simulink subsystem "Controller"  (R2021a)
settings: Solver=VariableStepAuto  StartTime=0.0  StopTime=10.0  RelTol=1e-3
values from neighbouring files (symbols this model uses):
  MPC =     [matlab.mat]
  N = [-39.9215617836 -39.7361560536 -39.4691718024 -38.8907059248 -38.267742672 -37.9562610456 -37.5112872936 -37.2888004176 -36.7993292904 -36.4433502888 -35.8648844112 -35.1974237832 ... (201 elements, 201x1)]    [matlab.mat]
  physics =     [matlab.mat]
  PWM = [1100 1104 1108 1112 1116 1120 1124 1128 1132 1136 1140 1144 ... (201 elements, 201x1)]    [matlab.mat]
libraries: mpclib x5, sharedTrackingLibrary x3, sharedtransform x2, simulink x1
settings Model: Creator=Lamarre  LastModifiedBy=lamarre
settings SolverCC: AlgebraicLoopSolver=TrustRegion
settings DebuggingCC: SFMachineParentedDataDiag=warning

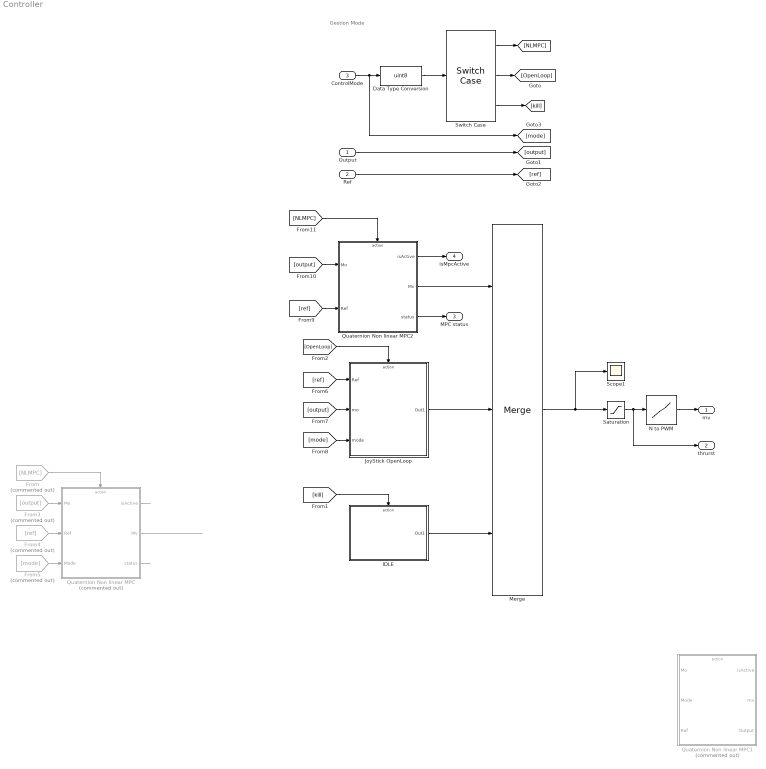
== system Controller ==
  note: Gestion Mode
  Output : Inport
  Ref : Inport  Port=2
  ControlMode : Inport  Port=3
  Data Type Conversion : DataTypeConversion  OutDataTypeStr=uint8
  From : From  Commented=on  GotoTag=NLMPC
  From3 : From  Commented=on  GotoTag=output
  From4 : From  Commented=on  GotoTag=ref
  From5 : From  Commented=on  GotoTag=mode
  IDLE : Subsystem  TreatAsAtomicUnit=on
  JoyStick OpenLoop : Subsystem  TreatAsAtomicUnit=on
  Merge : Merge  Inputs=3
  N to PWM : Lookup_n-D  NumberOfTableDimensions=1  BreakpointsForDimension1=N  BeginIndexSearchUsingPreviousIndexResult=on  Table=PWM  InterpMethod=Nearest  ExtrapMethod=Clip  DiagnosticForOutOfRangeInput=Warning  RemoveProtectionInput=on  InternalRulePriority=Speed  OutDataTypeStr=uint16  RndMeth=Simplest  InputSameDT=on
  Quaternion Non linear MPC : Subsystem  Commented=on
  Quaternion Non linear MPC1 : Subsystem  Commented=on
  Quaternion Non linear MPC2 : Subsystem
  Saturation : Saturate  UpperLimit=MPC.tmax  LowerLimit=MPC.tmin
  Scope1 : Scope
  Switch Case : SwitchCase  CaseConditions={mpcMode, openLoopMode}
  mv : Outport
  thrurst : Outport  Port=2
  MPC status : Outport  Port=3
  isMpcActive : Outport  Port=4
  wires:
  Switch Case/3 -> [kill]
  Switch Case/1 -> [NLMPC]
  N to PWM/1 -> mv/1
  [kill] -> IDLE/Action
  Data Type Conversion/1 -> Switch Case/1
  Switch Case/2 -> [OpenLoop]
  JoyStick OpenLoop/1(Out1) -> Merge/2
  IDLE/1(Out1) -> Merge/3
  [OpenLoop] -> JoyStick OpenLoop/Action
  ControlMode/1 -> Data Type Conversion/1, [mode]
  Output/1 -> [output]
  Ref/1 -> [ref]
  [ref] -> JoyStick OpenLoop/1(Ref)
  [output] -> JoyStick OpenLoop/2(mo)
  [mode] -> JoyStick OpenLoop/3(mode)
  Saturation/1 -> N to PWM/1, thrurst/1
  Merge/1 -> Scope1/1, Saturation/1
  [output] -> Quaternion Non linear MPC2/1(Mo)
  [ref] -> Quaternion Non linear MPC2/2(Ref)
  From3/1 -> Quaternion Non linear MPC/1(Mo)
  Quaternion Non linear MPC/3(status) -> ?
  From4/1 -> Quaternion Non linear MPC/2(Ref)
  From5/1 -> Quaternion Non linear MPC/3(Mode)
  Quaternion Non linear MPC/1(isActive) -> ?
  From/1 -> Quaternion Non linear MPC/Action
  Quaternion Non linear MPC/2(Mv) -> ?
  Quaternion Non linear MPC2/3(status) -> MPC status/1
  Quaternion Non linear MPC2/1(isActive) -> isMpcActive/1
  Quaternion Non linear MPC2/2(Mv) -> Merge/1
  [NLMPC] -> Quaternion Non linear MPC2/Action

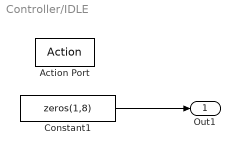
== system Controller/IDLE ==
  Action Port : ActionPort
  Constant1 : Constant  Value=zeros(1,8)
  Out1 : Outport
  wires:
  Constant1/1 -> Out1/1

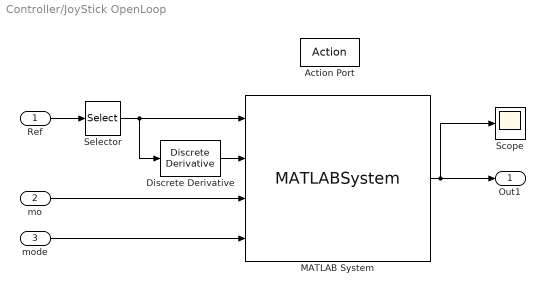
== system Controller/JoyStick OpenLoop ==
  Ref : Inport
  mo : Inport  Port=2
  mode : Inport  Port=3
  Action Port : ActionPort
  Discrete Derivative : simulink/Discrete/Discrete Derivative  gainval=1.0  ICPrevScaledInput=0.0  OutMin=[]  OutMax=[]  OutDataType=fixdt(1, 16)  OutScaling=2^-10  DoSatur=off
  MATLAB System : MATLABSystem  System=OpenLoopController  k=40  binv=binv  mass=physics.mass  volume=physics.volume  height=physics.height  I=physics.I  RG=physics.RG  RB=physics.RB  AddedMass=physics.AddedMass  CDL=physics.CDL  CDQ=physics.CDQ  AF=physics.AF  g=physics.g  rho=physics.rho  SimulateUsing=Code generation
      mask Type: OpenLoopController
      mask Display:
      | disp('OpenLoopController');
      | port_label('input',1,'ref');
      | port_label('input',2,'ref_dot');
      | port_label('input',3,'mo');
      | port_label('input',4,'mode');
      | port_label('output',1,'mv');
  Scope : Scope
  Selector : Selector  NumberOfDimensions=2  InputPortWidth=13  IndexOptions=Index vector (dialog),Index vector (dialog)  Indices=1,[8:13]  OutputSizes=1,1
  Out1 : Outport
  wires:
  Selector/1 -> MATLAB System/1, Discrete Derivative/1
  Discrete Derivative/1 -> MATLAB System/2
  Ref/1 -> Selector/1
  MATLAB System/1 -> Out1/1, Scope/1
  mode/1 -> MATLAB System/4
  mo/1 -> MATLAB System/3

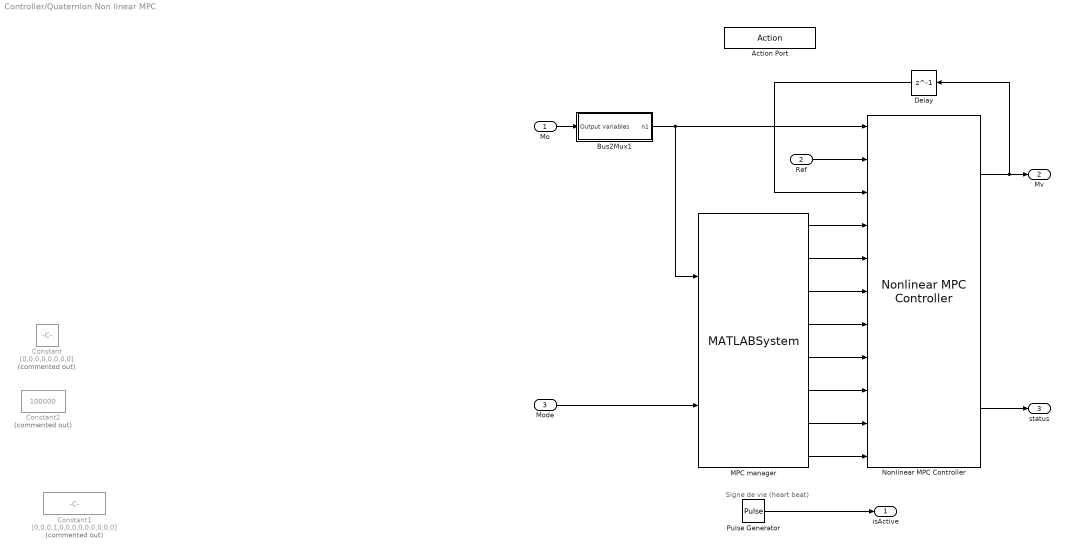
== system Controller/Quaternion Non linear MPC ==
  note: Signe de vie (heart beat)
  Mo : Inport
  Ref : Inport  Port=2
  Mode : Inport  Port=3
  Action Port : ActionPort  InitializeStates=reset
  Bus2Mux1 : Subsystem
  Constant : Constant  Commented=on  Value=[0,0,0,0,0,0,0,0]  VectorParams1D=off
  Constant1 : Constant  Commented=on  Value=[0,0,0,1,0,0,0,0,0,0,0,0,0]  VectorParams1D=off
  Constant2 : Constant  Commented=on  Value=100000
  Delay : Delay  DelayLength=1  InitialCondition=[0,0,0,0,0,0,0,0].'
  MPC manager : MATLABSystem  System=mpcManager  Config10=Config10  Config19=Config19  Tmin=ones( 1, 8 )*MPC.tmin  Tmax=ones( 1, 8 )*MPC.tmax  MecConst=constValues  mvInit=Ui  eInit=0  SimulateUsing=Code generation
      mask Type: mpcManager
      mask Display:
      | disp('mpcManager');
      | port_label('input',1,'x0');
      | port_label('input',2,'mode');
      | port_label('output',1,'mvmin');
      | port_label('output',2,'mvmax');
      | port_label('output',3,'ywt');
      | port_label('output',4,'mvwt');
      | port_label('output',5,'dmwwt');
      | port_label('output',6,'mvInit');
      | port_label('output',7,'xInit');
      | port_label('output',8,'eInit');
  Nonlinear MPC Controller : mpclib/Nonlinear MPC Controller  SCDEnableBlockLinearizationSpecification=on  nlmpcobj=nlobj  UseObjectTs=on  TsControl=mpc.Ts  UseMEX=off  md_enabled=off  mvtarget_enabled=off  param_enabled=off  cost_enabled=off  mvseq_enabled=off  stateseq_enabled=on  ovseq_enabled=off  slack_enabled=off  status_enabled=on  ov_min=off  ov_max=off  mv_min=on  mv_max=on  mvrate_min=off  mvrate_max=off  state_min=off  state_max=off  ov_weight=on  mv_weight=on  mvrate_weight=on  ecr_weight=off  nlp_initialize=on
  Pulse Generator : DiscretePulseGenerator  SampleTime=MPC.Ts
  isActive : Outport
  Mv : Outport  Port=2
  status : Outport  Port=3
  wires:
  Delay/1 -> Nonlinear MPC Controller/3
  Ref/1 -> Nonlinear MPC Controller/2
  Nonlinear MPC Controller/3 -> status/1
  MPC manager/8 -> Nonlinear MPC Controller/11
  MPC manager/7 -> Nonlinear MPC Controller/10
  MPC manager/5 -> Nonlinear MPC Controller/8
  MPC manager/6 -> Nonlinear MPC Controller/9
  MPC manager/4 -> Nonlinear MPC Controller/7
  MPC manager/3 -> Nonlinear MPC Controller/6
  MPC manager/2 -> Nonlinear MPC Controller/5
  MPC manager/1 -> Nonlinear MPC Controller/4
  Nonlinear MPC Controller/1 -> Delay/1, Mv/1
  Bus2Mux1/1(n1) -> MPC manager/1, Nonlinear MPC Controller/1
  Mode/1 -> MPC manager/2
  Pulse Generator/1 -> isActive/1
  Mo/1 -> Bus2Mux1/1(Output variables)

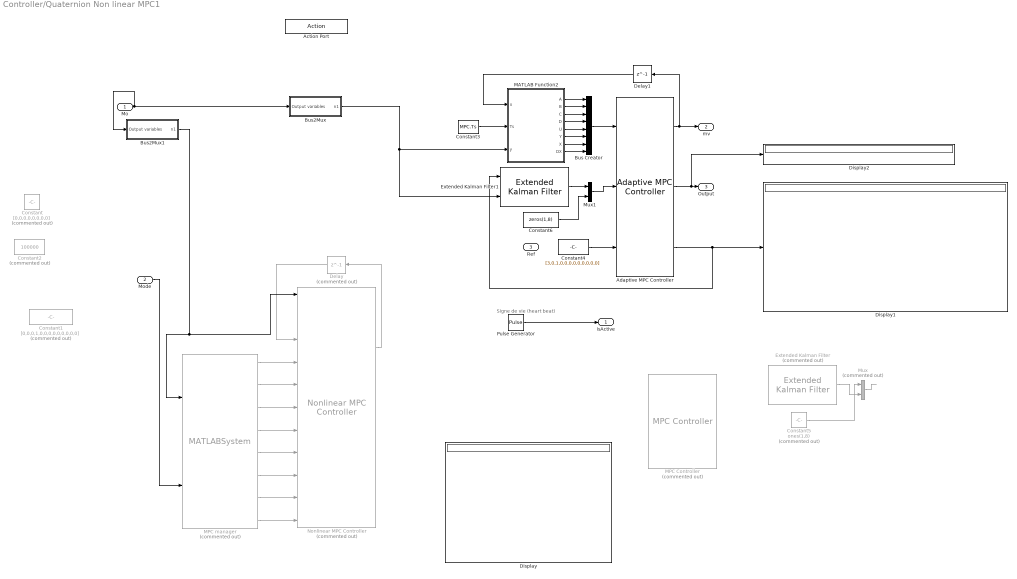
== system Controller/Quaternion Non linear MPC1 ==
  note: Signe de vie (heart beat)
  Mo : Inport
  Mode : Inport  Port=2
  Ref : Inport  Port=3
  Action Port : ActionPort  InitializeStates=reset
  Adaptive MPC Controller : mpclib/Adaptive MPC Controller  SCDEnableBlockLinearizationSpecification=on  mpcobj=mpcobj  x0=xss  enable_value=0  updateMPCinCallerWorkspace=on  md_inport=off  mv_inport=off  uref_inport=off  return_cost=off  return_mvseq=off  return_qpstatus=on  return_xseq=off  return_state=on  return_ovseq=off  state_inport=on  isltv_plant=off  umin_inport=off  umax_inport=off  ymin_inport=off  ymax_inport=off  cc_inport=off  ywt_inport=off  uwt_inport=off  duwt_inport=off  rhoeps_inport=off  pm_inport=off  MaximumP=10  HorizonChoice=FixedHorizon  BlockDataType=double  SampleTimeInherited=off  switch_inport=off
  Bus Creator : BusCreator  Inputs=8
  Bus2Mux : Subsystem
  Bus2Mux1 : Subsystem
  Constant : Constant  Commented=on  Value=[0,0,0,0,0,0,0,0]  VectorParams1D=off
  Constant1 : Constant  Commented=on  Value=[0,0,0,1,0,0,0,0,0,0,0,0,0]  VectorParams1D=off
  Constant2 : Constant  Commented=on  Value=100000
  Constant3 : Constant  Value=MPC.Ts
  Constant4 : Constant  Value=[3,0,1,0,0,0,0,0,0,0,0,0]  VectorParams1D=off
  Constant5 : Constant  Commented=on  Value=ones(1,8)
  Constant6 : Constant  Value=zeros(1,8)
  Delay : Delay  Commented=on  DelayLength=1  InitialCondition=[0,0,0,0,0,0,0,0].'
  Delay1 : Delay  DelayLength=1  InitialCondition=[0,0,0,0,0,0,0,0].'  SampleTime=.1
  Display : Display
  Display1 : Display
  Display2 : Display
  Extended Kalman Filter : sharedTrackingLibrary/Extended Kalman Filter  Commented=on  StateTransitionFcn=KalmanStateFonction  HasStateTransitionJacobianFcn=on  StateTransitionJacobianFcn=AUVQuatDiscreteJacobianMatrix  HasAdditiveProcessNoise=Additive  ProcessNoise=1  HasTimeVaryingProcessNoise=off  HasStateTransitionFcnExtraArgument=1  InitialState=[0,0,0.31,1,0,0,0,0,0,0,0,0,0]  InitialStateCovariance=1  MeasurementFcn1=KalmanMesuredFonction  HasMeasurementJacobianFcn1=off  HasMeasurementEnablePort1=off  HasAdditiveMeasurementNoise1=Additive  MeasurementNoise1=[1,1,1,1,1,1,1,1,1,1,1,1,1]  HasTimeVaryingMeasurementNoise1=off  HasMeasurementFcnExtraArgument1=0  MeasurementFcn2=myMeasurementFcn  HasMeasurementJacobianFcn2=off  HasMeasurementEnablePort2=off  HasAdditiveMeasurementNoise2=Nonadditive  MeasurementNoise2=1  HasTimeVaryingMeasurementNoise2=off  HasMeasurementFcnExtraArgument2=0  MeasurementFcn3=myMeasurementFcn  HasMeasurementJacobianFcn3=off  HasMeasurementEnablePort3=off  HasAdditiveMeasurementNoise3=Additive  MeasurementNoise3=1  HasTimeVaryingMeasurementNoise3=off  HasMeasurementFcnExtraArgument3=0  MeasurementFcn4=myMeasurementFcn  HasMeasurementJacobianFcn4=off  HasMeasurementEnablePort4=off  HasAdditiveMeasurementNoise4=Additive  MeasurementNoise4=1  HasTimeVaryingMeasurementNoise4=off  HasMeasurementFcnExtraArgument4=0  MeasurementFcn5=myMeasurementFcn  HasMeasurementJacobianFcn5=off  HasMeasurementEnablePort5=off  HasAdditiveMeasurementNoise5=Additive  MeasurementNoise5=1  HasTimeVaryingMeasurementNoise5=off  HasMeasurementFcnExtraArgument5=0  EnableMultirate=off  StateTransitionFcnSampleTime=1  MeasurementFcn1SampleTime=1  MeasurementFcn2SampleTime=1  MeasurementFcn3SampleTime=1  MeasurementFcn4SampleTime=1  MeasurementFcn5SampleTime=1  UseCurrentEstimator=on  OutputStateCovariance=off  DataType=double  SampleTime=MPC.Ts  NumberOfMeasurements=1
      settings: SourceProductBaseCode=CT,DR,TF,ID,LP,NV,AR,RO,RR,UV,VE
  Extended Kalman Filter1 : sharedTrackingLibrary/Extended Kalman Filter  StateTransitionFcn=KalmanStateFonction  HasStateTransitionJacobianFcn=on  StateTransitionJacobianFcn=AUVQuatDiscreteJacobianMatrix  HasAdditiveProcessNoise=Additive  ProcessNoise=1  HasTimeVaryingProcessNoise=off  HasStateTransitionFcnExtraArgument=1  InitialState=[0,0,0.31,0,0,0,0,0,0,0,0,0]  InitialStateCovariance=1  MeasurementFcn1=KalmanMesuredFonction  HasMeasurementJacobianFcn1=off  HasMeasurementEnablePort1=off  HasAdditiveMeasurementNoise1=Additive  MeasurementNoise1=[1,1,1,1,1,1,1,1,1,1,1,1]  HasTimeVaryingMeasurementNoise1=off  HasMeasurementFcnExtraArgument1=0  MeasurementFcn2=myMeasurementFcn  HasMeasurementJacobianFcn2=off  HasMeasurementEnablePort2=off  HasAdditiveMeasurementNoise2=Nonadditive  MeasurementNoise2=1  HasTimeVaryingMeasurementNoise2=off  HasMeasurementFcnExtraArgument2=0  MeasurementFcn3=myMeasurementFcn  HasMeasurementJacobianFcn3=off  HasMeasurementEnablePort3=off  HasAdditiveMeasurementNoise3=Additive  MeasurementNoise3=1  HasTimeVaryingMeasurementNoise3=off  HasMeasurementFcnExtraArgument3=0  MeasurementFcn4=myMeasurementFcn  HasMeasurementJacobianFcn4=off  HasMeasurementEnablePort4=off  HasAdditiveMeasurementNoise4=Additive  MeasurementNoise4=1  HasTimeVaryingMeasurementNoise4=off  HasMeasurementFcnExtraArgument4=0  MeasurementFcn5=myMeasurementFcn  HasMeasurementJacobianFcn5=off  HasMeasurementEnablePort5=off  HasAdditiveMeasurementNoise5=Additive  MeasurementNoise5=1  HasTimeVaryingMeasurementNoise5=off  HasMeasurementFcnExtraArgument5=0  EnableMultirate=off  StateTransitionFcnSampleTime=1  MeasurementFcn1SampleTime=1  MeasurementFcn2SampleTime=1  MeasurementFcn3SampleTime=1  MeasurementFcn4SampleTime=1  MeasurementFcn5SampleTime=1  UseCurrentEstimator=on  OutputStateCovariance=off  DataType=double  SampleTime=MPC.Ts  NumberOfMeasurements=1
      settings: SourceProductBaseCode=CT,DR,TF,ID,LP,NV,AR,RO,RR,UV,VE
  MATLAB Function2 : MATLAB Function  TreatAsAtomicUnit=on  SystemSampleTime=MPC.Ts
  MPC Controller : mpclib/MPC Controller  Commented=on  SCDEnableBlockLinearizationSpecification=on  mpcobj=mpcobj  x0=xss  is_multiple=0  enable_value=0  return_u0=off  updateMPCinCallerWorkspace=on  md_inport=off  mv_inport=off  uref_inport=off  return_cost=off  return_mvseq=off  return_qpstatus=off  return_xseq=off  return_state=off  return_ovseq=off  state_inport=off  umin_inport=off  umax_inport=off  ymin_inport=off  ymax_inport=off  cc_inport=off  ywt_inport=off  uwt_inport=off  duwt_inport=off  rhoeps_inport=off  pm_inport=off  MaximumP=10  HorizonChoice=FixedHorizon  n_ts=0.1  n_p=10  n_mv=8  n_md=0  n_ud=0  n_mo=12  n_uo=0  BlockDataType=double  SampleTimeInherited=off  switch_inport=off
  MPC manager : MATLABSystem  Commented=on  System=mpcManager  Config10=Config10  Config19=Config19  Tmin=ones( 1, 8 )*MPC.tmin  Tmax=ones( 1, 8 )*MPC.tmax  MecConst=constValues  mvInit=Ui  eInit=0  SimulateUsing=Code generation
      mask Type: mpcManager
      mask Display:
      | disp('mpcManager');
      | port_label('input',1,'x0');
      | port_label('input',2,'mode');
      | port_label('output',1,'mvmin');
      | port_label('output',2,'mvmax');
      | port_label('output',3,'ywt');
      | port_label('output',4,'mvwt');
      | port_label('output',5,'dmwwt');
      | port_label('output',6,'mvInit');
      | port_label('output',7,'xInit');
      | port_label('output',8,'eInit');
  Mux : Mux  Commented=on  Inputs=2
  Mux1 : Mux  Inputs=2
  Nonlinear MPC Controller : mpclib/Nonlinear MPC Controller  Commented=on  SCDEnableBlockLinearizationSpecification=on  nlmpcobj=nlobj  UseObjectTs=on  TsControl=mpc.Ts  UseMEX=off  md_enabled=off  mvtarget_enabled=off  param_enabled=off  cost_enabled=off  mvseq_enabled=off  stateseq_enabled=off  ovseq_enabled=off  slack_enabled=off  status_enabled=on  ov_min=off  ov_max=off  mv_min=on  mv_max=on  mvrate_min=off  mvrate_max=off  state_min=off  state_max=off  ov_weight=on  mv_weight=on  mvrate_weight=on  ecr_weight=off  nlp_initialize=on
  Pulse Generator : DiscretePulseGenerator  SampleTime=MPC.Ts
  isActive : Outport
  mv : Outport  Port=2
  Output : Outport  Port=3
  wires:
  Constant6/1 -> Mux1/2
  Mux1/1 -> Adaptive MPC Controller/2
  Extended Kalman Filter1/1 -> Mux1/1
  Adaptive MPC Controller/2 -> Output/1, Display2/1
  Adaptive MPC Controller/1 -> mv/1, Delay1/1
  Constant4/1 -> Adaptive MPC Controller/3
  Bus2Mux/1(n1) -> MATLAB Function2/3(y), Extended Kalman Filter1/2
  Mux/1 -> ?
  Extended Kalman Filter/1 -> Mux/2
  Constant5/1 -> Mux/1
  Adaptive MPC Controller/3 -> Display1/1, Extended Kalman Filter1/1
  MPC manager/8 -> Nonlinear MPC Controller/11
  MPC manager/7 -> Nonlinear MPC Controller/10
  MPC manager/5 -> Nonlinear MPC Controller/8
  MPC manager/6 -> Nonlinear MPC Controller/9
  MPC manager/4 -> Nonlinear MPC Controller/7
  MPC manager/3 -> Nonlinear MPC Controller/6
  MPC manager/2 -> Nonlinear MPC Controller/5
  MPC manager/1 -> Nonlinear MPC Controller/4
  MATLAB Function2/4(D) -> Bus Creator/4
  Constant3/1 -> MATLAB Function2/2(Ts)
  MATLAB Function2/5(U) -> Bus Creator/5
  MATLAB Function2/3(C) -> Bus Creator/3
  Delay1/1 -> MATLAB Function2/1(u)
  MATLAB Function2/8(DX) -> Bus Creator/8
  MATLAB Function2/2(B) -> Bus Creator/2
  Bus Creator/1 -> Adaptive MPC Controller/1
  MATLAB Function2/7(X) -> Bus Creator/7
  MATLAB Function2/6(Y) -> Bus Creator/6
  MATLAB Function2/1(A) -> Bus Creator/1
  Nonlinear MPC Controller/1 -> Delay/1
  Delay/1 -> Nonlinear MPC Controller/3
  Bus2Mux1/1(n1) -> Nonlinear MPC Controller/1, MPC manager/1
  Mode/1 -> MPC manager/2
  Pulse Generator/1 -> isActive/1
  Mo/1 -> Bus2Mux/1(Output variables), Bus2Mux1/1(Output variables)

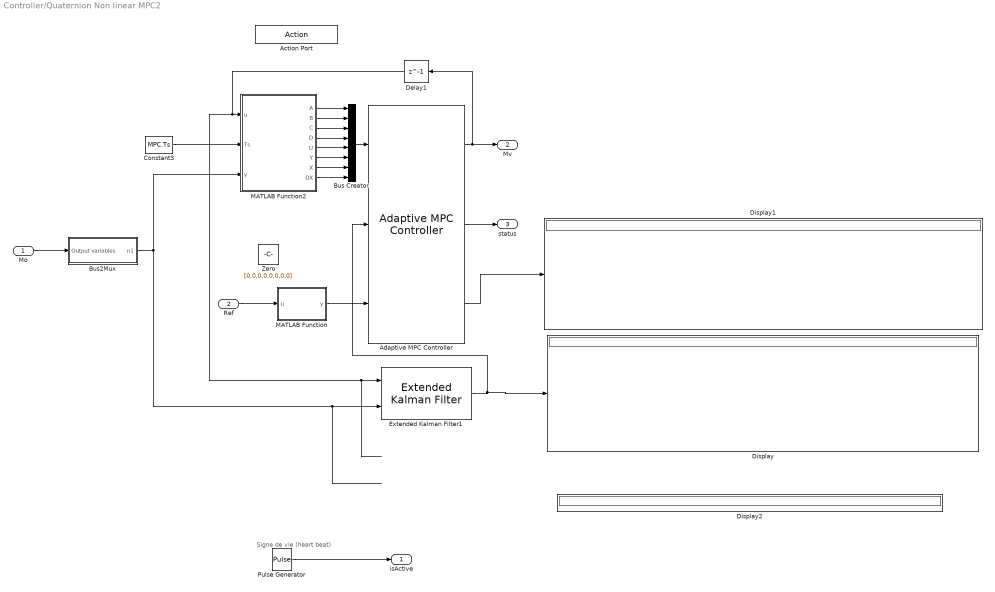
== system Controller/Quaternion Non linear MPC2 ==
  note: Signe de vie (heart beat)
  Mo : Inport
  Ref : Inport  Port=2
  Action Port : ActionPort  InitializeStates=reset
  Adaptive MPC Controller : mpclib/Adaptive MPC Controller  SCDEnableBlockLinearizationSpecification=on  mpcobj=mpcobj  enable_value=0  updateMPCinCallerWorkspace=on  md_inport=off  mv_inport=off  uref_inport=off  return_cost=off  return_mvseq=off  return_qpstatus=on  return_xseq=off  return_state=on  return_ovseq=off  state_inport=on  isltv_plant=off  umin_inport=off  umax_inport=off  ymin_inport=off  ymax_inport=off  cc_inport=off  ywt_inport=off  uwt_inport=off  duwt_inport=off  rhoeps_inport=off  pm_inport=off  MaximumP=10  HorizonChoice=FixedHorizon  BlockDataType=double  SampleTimeInherited=off  switch_inport=off
  Bus Creator : BusCreator  Inputs=8
  Bus2Mux : Subsystem
  Constant3 : Constant  Value=MPC.Ts
  Delay1 : Delay  DelayLength=1  InitialCondition=[0,0,0,0,0,0,0,0].'  SampleTime=.1
  Display : Display
  Display1 : Display
  Display2 : Display
  Extended Kalman Filter1 : sharedTrackingLibrary/Extended Kalman Filter  StateTransitionFcn=KalmanStateFonction  HasStateTransitionJacobianFcn=off  StateTransitionJacobianFcn=AUVQuatDiscreteJacobianMatrix  HasAdditiveProcessNoise=Additive  ProcessNoise=1  HasTimeVaryingProcessNoise=off  HasStateTransitionFcnExtraArgument=1  InitialState=[0,0,0.31,0,0,0,0,0,0,0,0,0,0,0,0,0,0,0,0,0]  InitialStateCovariance=1  MeasurementFcn1=KalmanMesuredFonction  HasMeasurementJacobianFcn1=off  HasMeasurementEnablePort1=off  HasAdditiveMeasurementNoise1=Additive  MeasurementNoise1=[1,1,1,1,1,1,1,1,1,1,1,1]  HasTimeVaryingMeasurementNoise1=off  HasMeasurementFcnExtraArgument1=0  MeasurementFcn2=myMeasurementFcn  HasMeasurementJacobianFcn2=off  HasMeasurementEnablePort2=off  HasAdditiveMeasurementNoise2=Nonadditive  MeasurementNoise2=1  HasTimeVaryingMeasurementNoise2=off  HasMeasurementFcnExtraArgument2=0  MeasurementFcn3=myMeasurementFcn  HasMeasurementJacobianFcn3=off  HasMeasurementEnablePort3=off  HasAdditiveMeasurementNoise3=Additive  MeasurementNoise3=1  HasTimeVaryingMeasurementNoise3=off  HasMeasurementFcnExtraArgument3=0  MeasurementFcn4=myMeasurementFcn  HasMeasurementJacobianFcn4=off  HasMeasurementEnablePort4=off  HasAdditiveMeasurementNoise4=Additive  MeasurementNoise4=1  HasTimeVaryingMeasurementNoise4=off  HasMeasurementFcnExtraArgument4=0  MeasurementFcn5=myMeasurementFcn  HasMeasurementJacobianFcn5=off  HasMeasurementEnablePort5=off  HasAdditiveMeasurementNoise5=Additive  MeasurementNoise5=1  HasTimeVaryingMeasurementNoise5=off  HasMeasurementFcnExtraArgument5=0  EnableMultirate=off  StateTransitionFcnSampleTime=1  MeasurementFcn1SampleTime=1  MeasurementFcn2SampleTime=1  MeasurementFcn3SampleTime=1  MeasurementFcn4SampleTime=1  MeasurementFcn5SampleTime=1  UseCurrentEstimator=on  OutputStateCovariance=off  DataType=double  SampleTime=MPC.Ts  NumberOfMeasurements=1
      settings: SourceProductBaseCode=CT,DR,TF,ID,LP,NV,AR,RO,RR,UV,VE
  MATLAB Function : MATLAB Function  TreatAsAtomicUnit=on
  MATLAB Function2 : MATLAB Function  TreatAsAtomicUnit=on  SystemSampleTime=MPC.Ts
  Pulse Generator : DiscretePulseGenerator  SampleTime=MPC.Ts
  Zero : Constant  Value=[0,0,0,0,0,0,0,0]  OutDataTypeStr=Inherit: Inherit via back propagation
  isActive : Outport
  Mv : Outport  Port=2
  status : Outport  Port=3
  wires:
  Extended Kalman Filter1/1 -> Adaptive MPC Controller/2, Display/1
  MATLAB Function/1(y) -> Adaptive MPC Controller/3
  Adaptive MPC Controller/3 -> Display1/1
  Bus2Mux/1(n1) -> Extended Kalman Filter1/2, MATLAB Function2/3(y)
  MATLAB Function2/7(X) -> Bus Creator/7
  Adaptive MPC Controller/2 -> status/1
  Ref/1 -> MATLAB Function/1(u)
  Constant3/1 -> MATLAB Function2/2(Ts)
  MATLAB Function2/6(Y) -> Bus Creator/6
  MATLAB Function2/1(A) -> Bus Creator/1
  MATLAB Function2/8(DX) -> Bus Creator/8
  MATLAB Function2/2(B) -> Bus Creator/2
  MATLAB Function2/5(U) -> Bus Creator/5
  Delay1/1 -> MATLAB Function2/1(u), Extended Kalman Filter1/1
  Bus Creator/1 -> Adaptive MPC Controller/1
  MATLAB Function2/3(C) -> Bus Creator/3
  MATLAB Function2/4(D) -> Bus Creator/4
  Adaptive MPC Controller/1 -> Delay1/1, Mv/1
  Pulse Generator/1 -> isActive/1
  Mo/1 -> Bus2Mux/1(Output variables)

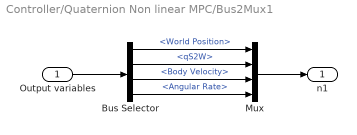
== system Controller/Quaternion Non linear MPC/Bus2Mux1 ==
  Output variables : Inport
  Bus Selector : BusSelector  OutputSignals=World Position,qS2W,Body Velocity,Angular Rate
  Mux : Mux
  n1 : Outport
  wires:
  Bus Selector/2 -> Mux/2  "<qS2W>"
  Bus Selector/3 -> Mux/3  "<Body Velocity>"
  Mux/1 -> n1/1
  Output variables/1 -> Bus Selector/1
  Bus Selector/4 -> Mux/4  "<Angular Rate>"
  Bus Selector/1 -> Mux/1  "<World Position>"

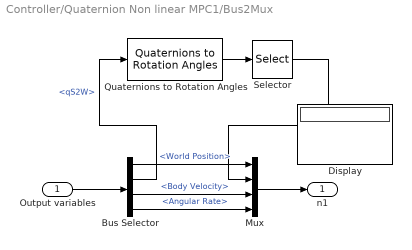
== system Controller/Quaternion Non linear MPC1/Bus2Mux ==
  Output variables : Inport
  Bus Selector : BusSelector  OutputSignals=World Position,qS2W,Body Velocity,Angular Rate
  Display : Display
  Mux : Mux
  Quaternions to Rotation Angles : sharedtransform/Quaternions to Rotation Angles  rotationOrder=ZYX  aMode=aMode
      settings: SourceProductBaseCode=AE,PW,DR,MT,UV,VE
  Selector : Selector  InputPortWidth=3  IndexOptions=Index vector (dialog)  Indices=[3,2,1]  OutputSizes=1
  n1 : Outport
  wires:
  Selector/1 -> Mux/2
  Quaternions to Rotation Angles/1 -> Selector/1
  Bus Selector/2 -> Quaternions to Rotation Angles/1  "<qS2W>"
  Bus Selector/3 -> Mux/3  "<Body Velocity>"
  Mux/1 -> n1/1
  Output variables/1 -> Bus Selector/1
  Bus Selector/4 -> Mux/4  "<Angular Rate>"
  Bus Selector/1 -> Mux/1  "<World Position>"

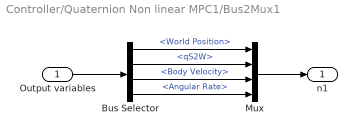
== system Controller/Quaternion Non linear MPC1/Bus2Mux1 ==
  Output variables : Inport
  Bus Selector : BusSelector  OutputSignals=World Position,qS2W,Body Velocity,Angular Rate
  Mux : Mux
  n1 : Outport
  wires:
  Bus Selector/2 -> Mux/2  "<qS2W>"
  Bus Selector/3 -> Mux/3  "<Body Velocity>"
  Mux/1 -> n1/1
  Output variables/1 -> Bus Selector/1
  Bus Selector/4 -> Mux/4  "<Angular Rate>"
  Bus Selector/1 -> Mux/1  "<World Position>"

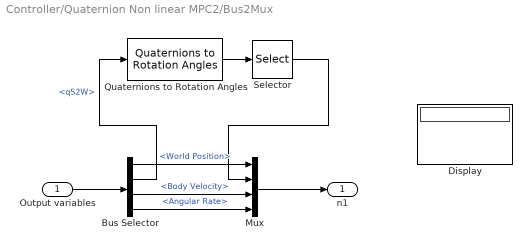
== system Controller/Quaternion Non linear MPC2/Bus2Mux ==
  Output variables : Inport
  Bus Selector : BusSelector  OutputSignals=World Position,qS2W,Body Velocity,Angular Rate
  Display : Display
  Mux : Mux
  Quaternions to Rotation Angles : sharedtransform/Quaternions to Rotation Angles  rotationOrder=ZYX  aMode=aMode
      settings: SourceProductBaseCode=AE,PW,DR,MT,UV,VE
  Selector : Selector  InputPortWidth=3  IndexOptions=Index vector (dialog)  Indices=[3,2,1]  OutputSizes=1
  n1 : Outport
  wires:
  Selector/1 -> Mux/2
  Quaternions to Rotation Angles/1 -> Selector/1
  Bus Selector/2 -> Quaternions to Rotation Angles/1  "<qS2W>"
  Bus Selector/3 -> Mux/3  "<Body Velocity>"
  Mux/1 -> n1/1
  Output variables/1 -> Bus Selector/1
  Bus Selector/4 -> Mux/4  "<Angular Rate>"
  Bus Selector/1 -> Mux/1  "<World Position>"

== matlab function Controller/Quaternion Non linear MPC2/MATLAB Function2 ==
  data: u input; Ts input; y input; A output; B output; C output; D output; U output; Y output; X output; DX output
function [A,B,C,D,U,Y,X,DX] = TrimPlant(u,Ts,y)
% Lineariser le model dynamique

[Ac, Bc, Cc, Dc]=AUVEULJacobianMatrix(y,u);
% Generate discrete-time model

nx = size(Ac,1);
nu = size(Bc,2);
M = expm([[Ac Bc]*Ts; zeros(nu,nu+nx)]);
A = M(1:nx,1:nx);
B = M(1:nx,nx+1:nx+nu);
C = Cc;
D = Dc;

% Nominal conditions for discrete-time plant
U=u.';
Y=(Cc*y + Dc*u).';
X=y.';
DX=(A*y+B*u-y).';

end

== matlab function Controller/Quaternion Non linear MPC1/MATLAB Function2 ==
  data: u input; Ts input; y input; A output; B output; C output; D output; U output; Y output; X output; DX output
function [A,B,C,D,U,Y,X,DX] = TrimPlant(u,Ts,y)
% Lineariser le model dynamique

[Ac, Bc, Cc, Dc]=AUVEULJacobianMatrix(y,u);
% Generate discrete-time model

nx = size(Ac,1);
nu = size(Bc,2);
M = expm([[Ac Bc]*Ts; zeros(nu,nu+nx)]);
A = M(1:nx,1:nx);
B = M(1:nx,nx+1:nx+nu);
C = Cc;
D = Dc;

% Nominal conditions for discrete-time plant
U=u.';
Y=(Cc*y + Dc*u).';
X=y.';
DX=(A*y+B*u-y).';

end

== matlab function Controller/Quaternion Non linear MPC2/MATLAB Function ==
  data: u input; y output size=[10,12]
function y = fcn(u)
    y=zeros(10,12);
    for i=1:10
        y(i,1:3) = u(i,1:3);
        y(i,4:6) = flip(quat2eul(u(i,4:7),'ZYX'));
        y(i,7:12)= u(i,8:13);       
    end    
end
